simulink model "test_d_v_p"  (Simulink 6.2)
settings: Solver=ode45  StartTime=0.0  StopTime=30000  RelTol=1e-3
undefined symbols (not defined in the file or in its folder): ant_bits, blockCountBits, blockRowBits
libraries: xbsIndex_r3 x843, xps_library x50, casper_library x17
(part 2 of 6)

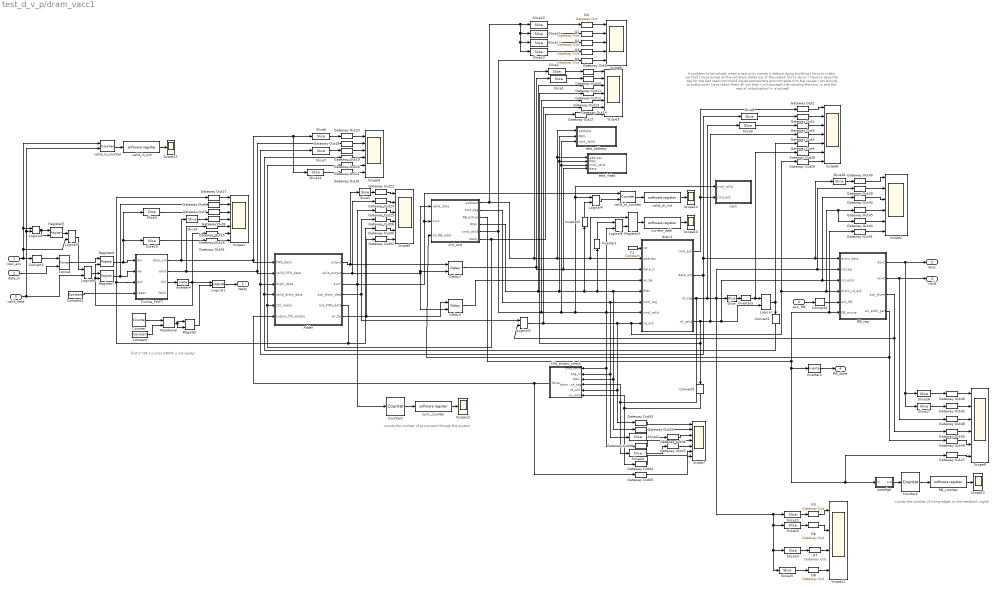
== system test_d_v_p/dram_vacc1 ==
  note: counts the number of rising edges on
      | the readback signal
  note: counts the number of syncs
      | sent through the system
  note: first 2^28-1 cycles DRAM
      | is not ready!
  note: A problem to be solved:
      | when a new sync comes in before doing anything I have to make sur
      | that I have acked all the old dram datas out of the output fifo
      | to do so: I have to save the tag for the last read command issued somewhere
      | and compare it to the values I am acking to make sure I have taken them all out
      | then I will proceed with sending the sync in and the rest of initialization!
      | it is solved!
  new_acc : Inport  Port=1  LatchInput=off
  data_in : Inport  Port=2  LatchInput=off
  valid_data : Inport  Port=3  LatchInput=off
  ack_RB : Inport  Port=4  LatchInput=off
  Adder : Subsystem
  C1 : xbsIndex_r3/Constant  const=0  equ=P=C  arith_type=Boolean  n_bits=1  bin_pt=0  opselect=C  inp2=PCIN>>17  opr=+  inp1=P  carry=CIN  iostate=0  explicit_period=on  period=1  dbl_ovrd=off
  Concat : xbsIndex_r3/Concat  num_inputs=2  explicit_period=off  period=1  dbl_ovrd=off
  Constant : xbsIndex_r3/Constant  const=2^28-1  equ=P=C  arith_type=Unsigned  n_bits=28  bin_pt=0  opselect=C  inp2=PCIN>>17  opr=+  inp1=P  carry=CIN  iostate=0  explicit_period=on  period=1  dbl_ovrd=off
  Constant1 : xbsIndex_r3/Constant  const=0  equ=P=C  arith_type=Boolean  n_bits=28  bin_pt=0  opselect=C  inp2=PCIN>>17  opr=+  inp1=P  carry=CIN  iostate=0  explicit_period=on  period=1  dbl_ovrd=off
  Convert1 : xbsIndex_r3/Convert  Orientation=down  arith_type=Boolean  n_bits=31  bin_pt=0  quantization=Truncate  overflow=Wrap  latency=0  explicit_period=off  period=1  dbl_ovrd=off  show_param=off  inserted_by_tool=off  pipeline=off
      settings: xl_area=[0, 0, 0, 0, 0, 0, 0]
  Convert2 : xbsIndex_r3/Convert  arith_type=Unsigned  n_bits=1  bin_pt=0  quantization=Truncate  overflow=Wrap  latency=0  explicit_period=off  period=1  dbl_ovrd=off  show_param=off  inserted_by_tool=off  pipeline=off
      settings: xl_area=[0, 0, 0, 0, 0, 0, 0]
  Convert3 : xbsIndex_r3/Convert  Orientation=down  arith_type=Boolean  n_bits=31  bin_pt=0  quantization=Truncate  overflow=Wrap  latency=0  explicit_period=off  period=1  dbl_ovrd=off  show_param=off  inserted_by_tool=off  pipeline=off
      settings: xl_area=[0, 0, 0, 0, 0, 0, 0]
  Convert4 : xbsIndex_r3/Convert  arith_type=Boolean  n_bits=31  bin_pt=0  quantization=Truncate  overflow=Wrap  latency=0  explicit_period=off  period=1  dbl_ovrd=off  show_param=off  inserted_by_tool=off  pipeline=off
      settings: xl_area=[0, 0, 0, 0, 0, 0, 0]
  Counter : xbsIndex_r3/Counter  cnt_type=Free Running  n_bits=28  bin_pt=0  arith_type=Unsigned  start_count=0  cnt_to=Inf  cnt_by_val=1  operation=Up  explicit_period=off  period=1  load_pin=off  rst=off  en=off  dbl_ovrd=off  show_param=off  use_rpm=on  gen_core=off
      settings: xl_area=[0, 0, 0, 0, 0, 0, 0]
  Counter1 : xbsIndex_r3/Counter  cnt_type=Free Running  n_bits=10  bin_pt=0  arith_type=Unsigned  start_count=0  cnt_to=Inf  cnt_by_val=1  operation=Up  explicit_period=off  period=1  load_pin=off  rst=off  en=on  dbl_ovrd=off  show_param=off  use_rpm=on  gen_core=off
      settings: xl_area=[0, 0, 0, 0, 0, 0, 0]
  Counter2 : xbsIndex_r3/Counter  cnt_type=Free Running  n_bits=10  bin_pt=0  arith_type=Unsigned  start_count=0  cnt_to=Inf  cnt_by_val=1  operation=Up  explicit_period=off  period=1  load_pin=off  rst=off  en=on  dbl_ovrd=off  show_param=off  use_rpm=on  gen_core=off
      settings: xl_area=[0, 0, 0, 0, 0, 0, 0]
  Delay1 : xbsIndex_r3/Delay  latency=1  reg_retiming=off  explicit_period=on  period=1  en=on  accept_only_valid=off  init_zero=on  dbl_ovrd=off  show_param=off
      settings: xl_area=[0, 0, 0, 0, 0, 0, 0]
  Delay2 : xbsIndex_r3/Delay  latency=1  reg_retiming=off  explicit_period=on  period=1  en=on  accept_only_valid=off  init_zero=on  dbl_ovrd=off  show_param=off
      settings: xl_area=[0, 0, 0, 0, 0, 0, 0]
  G{0..8} (9 alike) : xbsIndex_r3/Gateway Out  output_type=Double  nbits=8  bin_pt=6  arith_type=Boolean  quantization=Truncate  overflow=Wrap  hdl_port=off  timing_constraint=None  locs_specified=off  LOCs={}  needs_fixed_name=off  show_param=off
      settings: xl_area=[0, 0, 0, 0, 0, 0, 0]
  Gateway Out{1..52} (52 alike) : xbsIndex_r3/Gateway Out  output_type=Double  nbits=8  bin_pt=6  arith_type=Boolean  quantization=Truncate  overflow=Wrap  hdl_port=off  timing_constraint=None  locs_specified=off  LOCs={}  needs_fixed_name=off  show_param=off
      settings: xl_area=[0, 0, 0, 0, 0, 0, 0]
  Inverter1 : xbsIndex_r3/Inverter  Orientation=up  latency=0  explicit_period=off  period=1  en=off  dbl_ovrd=off  show_param=off
      settings: xl_area=[0, 0, 0, 0, 0, 0, 0]
  Inverter2 : xbsIndex_r3/Inverter  latency=0  explicit_period=off  period=1  en=off  dbl_ovrd=off  show_param=off
      settings: xl_area=[0, 0, 0, 0, 0, 0, 0]
  Inverter3 : xbsIndex_r3/Inverter  latency=0  explicit_period=off  period=1  en=off  dbl_ovrd=off  show_param=off
      settings: xl_area=[0, 0, 0, 0, 0, 0, 0]
  Inverter4 : xbsIndex_r3/Inverter  latency=0  explicit_period=off  period=1  en=off  dbl_ovrd=off  show_param=off
      settings: xl_area=[0, 0, 0, 0, 0, 0, 0]
  Inverter5 : xbsIndex_r3/Inverter  Orientation=up  latency=0  explicit_period=off  period=1  en=off  dbl_ovrd=off  show_param=off
      settings: xl_area=[0, 0, 0, 0, 0, 0, 0]
  Logical{,1,3..4,6,8} (6 alike) : xbsIndex_r3/Logical  logical_function=AND  inputs=2  precision=Full  arith_type=Unsigned  n_bits=8  bin_pt=2  align_bp=on  latency=0  explicit_period=off  period=1  en=off  dbl_ovrd=off  show_param=off
      settings: xl_area=[0, 0, 0, 0, 0, 0, 0]
  Logical2 : xbsIndex_r3/Logical  logical_function=OR  inputs=2  precision=Full  arith_type=Unsigned  n_bits=8  bin_pt=2  align_bp=on  latency=0  explicit_period=off  period=1  en=off  dbl_ovrd=off  show_param=off
      settings: xl_area=[0, 0, 0, 0, 0, 0, 0]
  Logical7 : xbsIndex_r3/Logical  logical_function=OR  inputs=2  precision=Full  arith_type=Unsigned  n_bits=8  bin_pt=2  align_bp=on  latency=0  explicit_period=off  period=1  en=off  dbl_ovrd=off  show_param=off
      settings: xl_area=[0, 0, 0, 0, 0, 0, 0]
  RB_counter : xps_library/software register  Tag=xps:sw_reg  io_dir=To Processor  arith_type=Unsigned  bitwidth=32  bin_pt=0  sample_period=1  gw_name=test_d_v_p_dram_vacc1_RB_counter_user_data_in
  RB_reg : Subsystem
  Register{,2,5..7} (5 alike) : xbsIndex_r3/Register  init=0  reg_only_valid=off  explicit_period=off  period=1  rst=off  en=on  out_en=off  dbl_ovrd=off  show_param=off
      settings: xl_area=[0, 0, 0, 0, 0, 0, 0]
  Relational : xbsIndex_r3/Relational  mode=a=b  latency=1  explicit_period=off  period=1  en=off  dbl_ovrd=off  show_param=off
      settings: xl_area=[0, 0, 0, 0, 0, 0, 0]
  Scope{1,3,7..8} (4 alike) : Scope  NumInputPorts=7
      Scope1 settings: TimeRange=30000  YMin=0~0~0.95~0.95~0~0.95~-1  YMax=1~1~1.05~1.05~1~1.05~1  SaveName=ScopeData7
      Scope3 settings: YMin=0~0~0~0~0~0~0  YMax=150~2500~1~1~1~1~1  SaveName=ScopeData6
      Scope7 settings: YMin=0~0~0~0~0~0.95~0  YMax=1~1100~7500~1~1~1.05~1  SaveName=ScopeData17
      Scope8 settings: YMin=0~0~2.68438e+008~0~0~0~0  YMax=1~11000~2.68439e+008~1~1~1~1  SaveName=ScopeData19
  Scope{10,12..15} (5 alike) : Scope
      Scope10 settings: YMin=0  YMax=100  SaveName=ScopeData27
      Scope12 settings: YMin=0  YMax=100  SaveName=ScopeData32
      Scope13 settings: YMin=0  YMax=100  SaveName=ScopeData33
      Scope14 settings: YMin=0  YMax=100  SaveName=ScopeData21
      Scope15 settings: YMin=0  YMax=100  SaveName=ScopeData24
  Scope11 : Scope  NumInputPorts=4
      settings: YMin=0~0.95~-1~1.9  YMax=120~1.05~1~2.1  SaveName=ScopeData28
  Scope{2,4..5,9} (4 alike) : Scope  NumInputPorts=6
      Scope2 settings: YMin=2.5~5e+008~0~0~0~0.95  YMax=12.5~2.75e+009~1~1~1~1.05  SaveName=ScopeData22
      Scope4 settings: YMin=0.95~0.95~-1~-1~0.95~-1  YMax=1.05~1.05~1~1~1.05~1  SaveName=ScopeData8
      Scope5 settings: YMin=0~0~-1~0~0~-5  YMax=250~1~1~1~1~5  SaveName=ScopeData9
      Scope9 settings: YMin=1.9~1.9~-1~0~-1~0.95  YMax=2.1~2.1~1~1~1~1.05  SaveName=ScopeData23
  Scope6 : Scope  NumInputPorts=5
      settings: YMin=0~0~0~0~0  YMax=200~4000~1~1~1  SaveName=ScopeData14
  Slice : xbsIndex_r3/Slice  mode=Upper Bit Location + Width  nbits=1  bit1=0  base1=MSB of Input  bit0=0  base0=LSB of Input  boolean_output=off  explicit_period=off  period=1  dbl_ovrd=off
  Slice{1,3..8,16..18} (10 alike) : xbsIndex_r3/Slice  mode=Lower Bit Location + Width  nbits=32  bit1=0  base1=MSB of Input  bit0=0  base0=LSB of Input  boolean_output=off  explicit_period=off  period=1  dbl_ovrd=off
  Slice{2,10,20,22} (4 alike) : xbsIndex_r3/Slice  mode=Lower Bit Location + Width  nbits=8  bit1=0  base1=MSB of Input  bit0=5  base0=LSB of Input  boolean_output=off  explicit_period=off  period=1  dbl_ovrd=off
  Slice11 : xbsIndex_r3/Slice  mode=Lower Bit Location + Width  nbits=14  bit1=0  base1=MSB of Input  bit0=14  base0=LSB of Input  boolean_output=off  explicit_period=off  period=1  dbl_ovrd=off
  Slice12 : xbsIndex_r3/Slice  mode=Lower Bit Location + Width  nbits=1  bit1=0  base1=MSB of Input  bit0=13  base0=LSB of Input  boolean_output=off  explicit_period=off  period=1  dbl_ovrd=off
  Slice13 : xbsIndex_r3/Slice  mode=Lower Bit Location + Width  nbits=2  bit1=0  base1=MSB of Input  bit0=28  base0=LSB of Input  boolean_output=off  explicit_period=off  period=1  dbl_ovrd=off
  Slice14 : xbsIndex_r3/Slice  mode=Upper Bit Location + Width  nbits=1  bit1=0  base1=MSB of Input  bit0=0  base0=LSB of Input  boolean_output=off  explicit_period=off  period=1  dbl_ovrd=off
  Slice19 : xbsIndex_r3/Slice  mode=Upper Bit Location + Width  nbits=1  bit1=0  base1=MSB of Input  bit0=0  base0=LSB of Input  boolean_output=off  explicit_period=off  period=1  dbl_ovrd=off
  Slice21 : xbsIndex_r3/Slice  mode=Lower Bit Location + Width  nbits=8  bit1=0  base1=MSB of Input  bit0=6  base0=LSB of Input  boolean_output=off  explicit_period=off  period=1  dbl_ovrd=off
  Slice23 : xbsIndex_r3/Slice  mode=Lower Bit Location + Width  nbits=14  bit1=0  base1=MSB of Input  bit0=15  base0=LSB of Input  boolean_output=off  explicit_period=off  period=1  dbl_ovrd=off
  Slice24 : xbsIndex_r3/Slice  mode=Lower Bit Location + Width  nbits=1  bit1=0  base1=MSB of Input  bit0=14  base0=LSB of Input  boolean_output=off  explicit_period=off  period=1  dbl_ovrd=off
  Slice25 : xbsIndex_r3/Slice  mode=Lower Bit Location + Width  nbits=2  bit1=0  base1=MSB of Input  bit0=29  base0=LSB of Input  boolean_output=off  explicit_period=off  period=1  dbl_ovrd=off
  Slice9 : xbsIndex_r3/Slice  mode=Lower Bit Location + Width  nbits=31  bit1=0  base1=MSB of Input  bit0=0  base0=LSB of Input  boolean_output=off  explicit_period=off  period=1  dbl_ovrd=off
  Trickle_FWFT : Subsystem  mask{depth=512}
      mask init:
      | cursys = gcb ; 
      | set_param([cursys, '/FIFO'], 'depth', depth);
      mask StyleString: popup(16|32|64|128|256|512|1K|2K|4K|8K|16K|32K|64K)
  cack : Subsystem
  ctrl_unit : Subsystem  mask{burst_length=valid_length, acc_length=acc_length}
      mask prompts: burst_length "Burst Length?"; acc_length "Accumulation length?"
  current_addr : xps_library/software register  Tag=xps:sw_reg  io_dir=To Processor  arith_type=Unsigned  bitwidth=32  bin_pt=0  sample_period=1  gw_name=test_d_v_p_dram_vacc1_current_addr_user_data_in
  dram1 : Subsystem  Tag=xps:dram  AncestorBlock=xps_library/dram  mask(dram){dimm=1, arith_type=Unsigned, bin_pt=0, ip_clock=200, sample_period=1, use_sim=on, bank_mgt=on, wide_data=off, half_burst=off, shared=on}
      mask prompts: arith_type "Data Type"; bin_pt "Data binary point"; ip_clock "Datapath clock rate (MHz)"; sample_period "Sample period"; use_sim "Simulate DRAM using ModelSim"; bank_mgt "Enable bank management"; wide_data "Use wide data bus (288 bits)"; half_burst "Use half-burst"; shared "Share with PowerPC"
      mask help:
      | Interface to 1GB DDR2 DIMMs on BEE2.
      |
      | To simulate using ModelSim, place a ModelSim block named 'ModelSim' (case-sensitive) in the top level of the design.
      mask init:
      | dram_mask;
      mask StyleString: popup(1|2|3|4),popup(Boolean|Unsigned|Signed  (2's comp)),edit,edit,edit,checkbox,checkbox,checkbox,checkbox,checkbox
      mask CallbackString:
      | |||||||myname=gcb;
      | if strcmp(get_param(myname, 'wide_data'), 'off')
      |     set_param(myname, 'MaskEnables', {'on','on','on','on','on','on','on','on','on','on'});
      | else
      |     set_param(myname, 'half_burst', 'off');
      |     set_param(myname, 'MaskEnables', {'on','on','on','on','on','on','on','on','off','on'});
      | end||
  fifo_empty_check : Subsystem  Orientation=left
  posedge : Subsystem
  sync_counter : xps_library/software register  Tag=xps:sw_reg  io_dir=To Processor  arith_type=Unsigned  bitwidth=32  bin_pt=0  sample_period=1  gw_name=test_d_v_p_dram_vacc1_sync_counter_user_data_in
  test_address : Subsystem
  test_index : Subsystem
  valid_dr_cnt : xps_library/software register  Tag=xps:sw_reg  io_dir=To Processor  arith_type=Unsigned  bitwidth=32  bin_pt=0  sample_period=1  gw_name=test_d_v_p_dram_vacc1_valid_dr_cnt_user_data_in
  valid_dr_counter : xbsIndex_r3/Counter  cnt_type=Count Limited  n_bits=32  bin_pt=0  arith_type=Unsigned  start_count=0  cnt_to=Inf  cnt_by_val=1  operation=Up  explicit_period=off  period=1  load_pin=off  rst=on  en=on  dbl_ovrd=off  show_param=off  use_rpm=on  gen_core=off
      settings: xl_area=[0, 0, 0, 0, 0, 0, 0]
  valid_in_cnt : xps_library/software register  Tag=xps:sw_reg  io_dir=To Processor  arith_type=Unsigned  bitwidth=32  bin_pt=0  sample_period=1  gw_name=test_d_v_p_dram_vacc1_valid_in_cnt_user_data_in
  valid_in_counter : xbsIndex_r3/Counter  cnt_type=Count Limited  n_bits=32  bin_pt=0  arith_type=Unsigned  start_count=0  cnt_to=Inf  cnt_by_val=1  operation=Up  explicit_period=off  period=1  load_pin=off  rst=on  en=on  dbl_ovrd=off  show_param=off  use_rpm=on  gen_core=off
      settings: xl_area=[0, 0, 0, 0, 0, 0, 0]
  ready : Outport
  dout : Outport  Port=2
  valid : Outport  Port=3
  RB_done : Outport  Port=4
  wires:
  Convert4/1 -> RB_reg/5(ack_RB)
  Inverter3/1 -> Gateway Out28/1, Logical/1
  ack_RB/1 -> Convert4/1
  ctrl_unit/5(cmd_valid) -> G4/1, Gateway Out13/1, Logical6/2, Gateway Out38/1, fifo_empty_check/1(cmd_valid), dram1/7(cmd_valid), cack/1(cmd_valid), Logical4/1, test_address/3(cmd_valid), test_index/3(cmd_valid)
  Inverter2/1 -> RB_done/1
  posedge/1(out) -> Counter2/1
  RB_counter/1 -> Scope13/1
  Counter2/1 -> RB_counter/1
  sync_counter/1 -> Scope12/1
  Counter1/1 -> sync_counter/1
  Inverter4/1 -> Logical1/1, Gateway Out16/1, Register7/2, Register6/2
  G8/1 -> Scope11/4
  G7/1 -> Scope11/3
  G6/1 -> Scope11/2
  G5/1 -> Scope11/1
  Slice25/1 -> G8/1
  Slice24/1 -> G7/1
  Slice23/1 -> G6/1
  Slice21/1 -> G5/1
  Slice20/1 -> Gateway Out37/1
  Slice22/1 -> Gateway Out36/1
  current_addr/1 -> Scope10/1
  Inverter1/1 -> Logical6/1
  Logical6/1 -> Register2/2
  Register2/1 -> current_addr/1
  Slice19/1 -> Gateway Out51/1
  Gateway Out51/1 -> Scope1/7
  Register7/1 -> Gateway Out6/1, Trickle_FWFT/2(we)
  Register/1 -> Logical1/2
  Relational/1 -> Register/2, Register/1
  Constant/1 -> Relational/2
  Counter/1 -> Relational/1
  Logical1/1 -> ready/1
  Gateway Out47/1 -> Scope9/6
  Slice18/1 -> Gateway Out40/1
  Slice17/1 -> Gateway Out42/1
  Slice16/1 -> Gateway Out46/1
  Convert3/1 -> Gateway Out34/1, fifo_empty_check/6(rd_valid)
  Gateway Out49/1 -> Scope9/5
  Gateway Out50/1 -> Scope9/4
  Gateway Out48/1 -> Scope9/3
  Gateway Out42/1 -> Scope9/2
  Gateway Out46/1 -> Scope9/1
  Gateway Out41/1 -> Scope2/6
  Gateway Out44/1 -> Scope2/5
  Gateway Out45/1 -> Scope2/4
  Gateway Out43/1 -> Scope2/3
  Gateway Out39/1 -> Scope2/2
  Gateway Out40/1 -> Scope2/1
  Logical2/1 -> Gateway Out14/1, Gateway Out44/1, Gateway Out45/1, RB_reg/4(dram_rd_ack), Gateway Out29/1, dram1/8(rd_ack), Gateway Out33/1, fifo_empty_check/5(rd_ack)
  ctrl_unit/3(RB_active) -> Inverter2/1, posedge/1(in), Gateway Out47/1, RB_reg/6(RB_active), Gateway Out41/1
  RB_reg/4(en_addr_gen) -> Gateway Out49/1, ctrl_unit/3(en_RB_addr)
  RB_reg/3(ack_dram) -> Logical2/2, Gateway Out50/1
  RB_reg/2(valid) -> valid/1, Gateway Out48/1
  RB_reg/1(dout) -> Slice17/1, Slice16/1, dout/1
  Gateway Out29/1 -> Scope8/7
  Gateway Out28/1 -> Scope8/6
  Gateway Out4/1 -> Scope8/5
  Gateway Out5/1 -> Scope8/4
  Gateway Out3/1 -> Scope8/3
  Gateway Out1/1 -> Scope8/2
  Gateway Out2/1 -> Scope8/1
  Gateway Out35/1 -> Scope7/7
  Gateway Out34/1 -> Scope7/6
  Gateway Out38/1 -> Scope7/4
  Gateway Out37/1 -> Scope7/5
  Gateway Out36/1 -> Scope7/3
  Gateway Out32/1 -> Scope7/2
  Gateway Out33/1 -> Scope7/1
  fifo_empty_check/1(done) -> Gateway Out35/1, Adder/6(output_fifo_empty)
  Delay1/1 -> Slice1/1, dram1/3(data_in), test_index/4(data)
  Slice14/1 -> Gateway Out31/1
  Gateway Out31/1 -> Scope4/6
  G4/1 -> Scope6/5
  G3/1 -> Scope6/4
  G2/1 -> Scope6/3
  G1/1 -> Scope6/2
  G0/1 -> Scope6/1
  Slice13/1 -> G3/1
  Slice12/1 -> G2/1
  Slice11/1 -> G1/1
  Slice10/1 -> G0/1
  Gateway Out30/1 -> Scope5/5
  Adder/5(ack_FIFO_data) -> Gateway Out30/1, Gateway Out17/1, Trickle_FWFT/3(ack)
  Slice9/1 -> Gateway Out3/1
  Slice8/1 -> Gateway Out1/1
  Gateway Out27/1 -> Scope3/7
  Slice7/1 -> Gateway Out19/1
  Slice6/1 -> Gateway Out23/1
  Slice5/1 -> Gateway Out22/1
  Convert1/1 -> Adder/4(valid_dram_data), Gateway Out20/1
  Slice4/1 -> Gateway Out8/1
  Slice3/1 -> Gateway Out7/1
  Gateway Out26/1 -> Scope5/4
  Gateway Out25/1 -> Scope5/3
  Gateway Out24/1 -> Scope5/2
  Gateway Out22/1 -> Scope5/1
  Gateway Out21/1 -> Scope4/5
  Gateway Out20/1 -> Scope4/4
  Gateway Out19/1 -> Scope4/3
  Gateway Out18/1 -> Scope4/2
  Gateway Out23/1 -> Scope4/1
  Gateway Out16/1 -> Scope1/6
  Gateway Out15/1 -> Scope1/5
  Gateway Out8/1 -> Scope1/4
  Gateway Out7/1 -> Scope1/3
  Gateway Out6/1 -> Scope1/2
  Gateway Out17/1 -> Scope1/1
  Slice2/1 -> Gateway Out9/1
  Slice1/1 -> Gateway Out10/1
  Gateway Out14/1 -> Scope3/6
  Gateway Out13/1 -> Scope3/5
  Gateway Out12/1 -> Scope3/4
  Gateway Out11/1 -> Scope3/3
  Gateway Out10/1 -> Scope3/2
  Gateway Out9/1 -> Scope3/1
  Register6/1 -> Slice19/1, Slice3/1, Trickle_FWFT/1(din)
  Trickle_FWFT/3(full) -> Inverter4/1
  ctrl_unit/2(cmd_tag) -> Slice22/1, fifo_empty_check/2(tag_in), dram1/6(cmd_tag)
  dram1/1(cmd_ack) -> Gateway Out2/1, cack/2(cmd_ack)
  Adder/3(sync) -> Counter1/1, ctrl_unit/2(sync), valid_dr_counter/1, Gateway Out25/1
  Adder/2(valid_output) -> Gateway Out24/1, Delay1/2, ctrl_unit/1(valid_data), Delay2/2
  ctrl_unit/6(ready) -> Gateway Out27/1, Adder/5(ctrl_ready), Gateway Out21/1
  Logical/1 -> Convert1/1, Gateway Out4/1
  dram1/4(rd_valid) -> Convert3/1, Gateway Out12/1, RB_reg/3(rd_valid), Gateway Out43/1, Logical/2, Gateway Out5/1
  Slice/1 -> Inverter3/1
  dram1/3(rd_tag) -> Slice20/1, fifo_empty_check/4(dram_data_tag), RB_reg/2(rd_tag), Gateway Out39/1, Slice/1, Slice24/1, Slice25/1, Slice23/1, Slice21/1, Slice9/1
  dram1/2(data_out) -> RB_reg/1(dram_data), Slice18/1, Slice8/1, Adder/3(dram_data), Slice7/1
  Adder/1(output) -> Delay1/1, Slice5/1
  C1/1 -> dram1/1(rst)
  ctrl_unit/4(RWn) -> Gateway Out11/1, Inverter1/1, Gateway Out32/1, fifo_empty_check/3(RWn), dram1/5(RWn), Inverter5/1, test_address/2(RWn), test_index/2(RWn)
  ctrl_unit/1(address) -> Slice2/1, Register2/1, dram1/2(address), test_address/1(address), test_index/1(address), Slice12/1, Slice13/1, Slice11/1, Slice10/1
  Trickle_FWFT/2(valid) -> Adder/2(valid_FIFO_data), Gateway Out18/1, Gateway Out15/1
  Trickle_FWFT/1(data_out) -> Slice4/1, Slice14/1, Slice6/1, Adder/1(FIFO_data)
  Adder/4(ack_dram_data) -> Logical2/1, Gateway Out26/1
  new_acc/1 -> Convert2/1, Logical7/2, Logical3/1, valid_in_counter/1
  data_in/1 -> Concat/2
  valid_data/1 -> Logical8/2, Logical3/2, valid_in_counter/2
  Convert2/1 -> Concat/1
  Register5/1 -> Logical7/1
  Logical7/1 -> Logical8/1
  Logical3/1 -> Register5/1, Register5/2
  Concat/1 -> Register6/1
  Logical8/1 -> Register7/1
  Constant1/1 -> Trickle_FWFT/4(reset)
  Logical4/1 -> valid_dr_counter/2
  valid_dr_cnt/1 -> Scope14/1
  valid_dr_counter/1 -> valid_dr_cnt/1
  Inverter5/1 -> Logical4/2
  valid_in_cnt/1 -> Scope15/1
  valid_in_counter/1 -> valid_in_cnt/1
  Adder/6(wr_be) -> Delay2/1, Gateway Out52/1
  Delay2/1 -> dram1/4(wr_be)
  Gateway Out52/1 -> Scope5/6

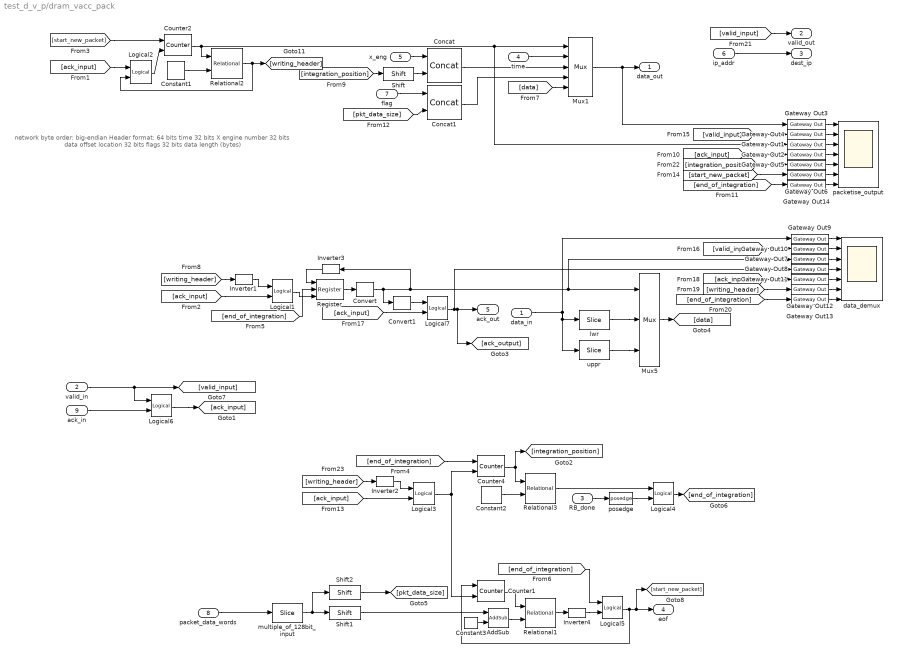
== system test_d_v_p/dram_vacc_pack ==
  note: network byte order: big-endian
      |
      | Header format:
      | 64 bits time
      | 32 bits X engine number
      | 32 bits data offset location
      | 32 bits flags
      | 32 bits data length (bytes)
  data_in : Inport  Port=1  LatchInput=off
  valid_in : Inport  Port=2  LatchInput=off
  RB_done : Inport  Port=3  LatchInput=off
  time : Inport  Port=4  LatchInput=off
  x_eng : Inport  Port=5  LatchInput=off
  ip_addr : Inport  Port=6  LatchInput=off
  flag : Inport  Port=7  LatchInput=off
  packet_data_words : Inport  Port=8  LatchInput=off
  ack_in : Inport  Port=9  LatchInput=off
  AddSub : xbsIndex_r3/AddSub  mode=Subtraction  precision=Full  arith_type=Unsigned  n_bits=8  bin_pt=2  quantization=Truncate  overflow=Wrap  latency=0  explicit_period=on  period=1  use_carryin=off  use_carryout=off  en=off  dbl_ovrd=off  show_param=off  use_core=on  pipeline=off  use_rpm=on  gen_core=off
      settings: xl_area=[0, 0, 0, 0, 0, 0, 0]
  Concat : xbsIndex_r3/Concat  num_inputs=2  explicit_period=off  period=1  dbl_ovrd=off
  Concat1 : xbsIndex_r3/Concat  num_inputs=2  explicit_period=off  period=1  dbl_ovrd=off
  Constant1 : xbsIndex_r3/Constant  const=2  equ=P=C  arith_type=Unsigned  n_bits=2  bin_pt=0  opselect=C  inp2=PCIN>>17  opr=+  inp1=P  carry=CIN  iostate=0  explicit_period=off  period=1  dbl_ovrd=off
  Constant2 : xbsIndex_r3/Constant  const=2*vector_len-1  equ=P=C  arith_type=Unsigned  n_bits=32  bin_pt=0  opselect=C  inp2=PCIN>>17  opr=+  inp1=P  carry=CIN  iostate=0  explicit_period=off  period=1  dbl_ovrd=off
  Constant3 : xbsIndex_r3/Constant  const=2  equ=P=C  arith_type=Unsigned  n_bits=32  bin_pt=0  opselect=C  inp2=PCIN>>17  opr=+  inp1=P  carry=CIN  iostate=0  explicit_period=off  period=1  dbl_ovrd=off
  Convert : xbsIndex_r3/Convert  arith_type=Unsigned  n_bits=1  bin_pt=0  quantization=Truncate  overflow=Wrap  latency=0  explicit_period=off  period=1  dbl_ovrd=off  show_param=off  inserted_by_tool=off  pipeline=off
      settings: xl_area=[0, 0, 0, 0, 0, 0, 0]
  Convert1 : xbsIndex_r3/Convert  arith_type=Boolean  n_bits=1  bin_pt=0  quantization=Truncate  overflow=Wrap  latency=0  explicit_period=off  period=1  dbl_ovrd=off  show_param=off  inserted_by_tool=off  pipeline=off
      settings: xl_area=[0, 0, 0, 0, 0, 0, 0]
  Counter1 : xbsIndex_r3/Counter  cnt_type=Free Running  n_bits=32  bin_pt=0  arith_type=Unsigned  start_count=0  cnt_to=1023  cnt_by_val=1  operation=Up  explicit_period=on  period=1  load_pin=off  rst=on  en=on  dbl_ovrd=off  show_param=off  use_rpm=on  gen_core=off
      settings: xl_area=[0, 0, 0, 0, 0, 0, 0]
  Counter2 : xbsIndex_r3/Counter  cnt_type=Free Running  n_bits=2  bin_pt=0  arith_type=Unsigned  start_count=0  cnt_to=1023  cnt_by_val=1  operation=Up  explicit_period=on  period=1  load_pin=off  rst=on  en=on  dbl_ovrd=off  show_param=off  use_rpm=on  gen_core=off
      settings: xl_area=[0, 0, 0, 0, 0, 0, 0]
  Counter4 : xbsIndex_r3/Counter  cnt_type=Free Running  n_bits=32  bin_pt=0  arith_type=Unsigned  start_count=0  cnt_to=1023  cnt_by_val=1  operation=Up  explicit_period=on  period=1  load_pin=off  rst=on  en=on  dbl_ovrd=off  show_param=off  use_rpm=on  gen_core=off
      settings: xl_area=[0, 0, 0, 0, 0, 0, 0]
  Gateway Out{1..14} (14 alike) : xbsIndex_r3/Gateway Out  output_type=Double  nbits=8  bin_pt=6  arith_type=Boolean  quantization=Truncate  overflow=Wrap  hdl_port=on  timing_constraint=None  locs_specified=off  LOCs={}  needs_fixed_name=off  show_param=off
      settings: xl_area=[0, 0, 0, 0, 0, 0, 0]
  Inverter1 : xbsIndex_r3/Inverter  latency=0  explicit_period=off  period=1  en=off  dbl_ovrd=off  show_param=off
      settings: xl_area=[0, 0, 0, 0, 0, 0, 0]
  Inverter2 : xbsIndex_r3/Inverter  latency=0  explicit_period=off  period=1  en=off  dbl_ovrd=off  show_param=off
      settings: xl_area=[0, 0, 0, 0, 0, 0, 0]
  Inverter3 : xbsIndex_r3/Inverter  Orientation=left  latency=0  explicit_period=on  period=1  en=off  dbl_ovrd=off  show_param=off
      settings: xl_area=[0, 0, 0, 0, 0, 0, 0]
  Inverter4 : xbsIndex_r3/Inverter  latency=0  explicit_period=off  period=1  en=off  dbl_ovrd=off  show_param=off
      settings: xl_area=[0, 0, 0, 0, 0, 0, 0]
  Logical{1..3,6..7} (5 alike) : xbsIndex_r3/Logical  logical_function=AND  inputs=2  precision=Full  arith_type=Unsigned  n_bits=8  bin_pt=2  align_bp=on  latency=0  explicit_period=off  period=1  en=off  dbl_ovrd=off  show_param=off
      settings: xl_area=[0, 0, 0, 0, 0, 0, 0]
  Logical4 : xbsIndex_r3/Logical  logical_function=OR  inputs=2  precision=Full  arith_type=Unsigned  n_bits=8  bin_pt=2  align_bp=on  latency=0  explicit_period=off  period=1  en=off  dbl_ovrd=off  show_param=off
      settings: xl_area=[0, 0, 0, 0, 0, 0, 0]
  Logical5 : xbsIndex_r3/Logical  logical_function=OR  inputs=2  precision=Full  arith_type=Unsigned  n_bits=8  bin_pt=2  align_bp=on  latency=0  explicit_period=off  period=1  en=off  dbl_ovrd=off  show_param=off
      settings: xl_area=[0, 0, 0, 0, 0, 0, 0]
  Mux1 : xbsIndex_r3/Mux  inputs=4  precision=Full  arith_type="Signed  (2's comp)"  n_bits=8  bin_pt=2  quantization=Truncate  overflow=Wrap  latency=0  explicit_period=off  period=1  en=off  dbl_ovrd=off  show_param=off  mux_type=off  use_rpm=off  gen_core=off
      settings: xl_area=[0, 0, 0, 0, 0, 0, 0]
  Mux5 : xbsIndex_r3/Mux  inputs=2  precision=Full  arith_type="Signed  (2's comp)"  n_bits=8  bin_pt=2  quantization=Truncate  overflow=Wrap  latency=0  explicit_period=on  period=1  en=off  dbl_ovrd=off  show_param=off  mux_type=off  use_rpm=off  gen_core=off
      settings: xl_area=[0, 0, 0, 0, 0, 0, 0]
  Register : xbsIndex_r3/Register  init=0  reg_only_valid=off  explicit_period=on  period=1  rst=on  en=on  out_en=off  dbl_ovrd=off  show_param=off
      settings: xl_area=[0, 0, 0, 0, 0, 0, 0]
  Relational1 : xbsIndex_r3/Relational  mode=a<=b  latency=0  explicit_period=off  period=1  en=off  dbl_ovrd=off  show_param=off
      settings: xl_area=[0, 0, 0, 0, 0, 0, 0]
  Relational2 : xbsIndex_r3/Relational  mode=a<=b  latency=0  explicit_period=off  period=1  en=off  dbl_ovrd=off  show_param=off
      settings: xl_area=[0, 0, 0, 0, 0, 0, 0]
  Relational3 : xbsIndex_r3/Relational  mode=a>=b  latency=0  explicit_period=off  period=1  en=off  dbl_ovrd=off  show_param=off
      settings: xl_area=[0, 0, 0, 0, 0, 0, 0]
  Shift : xbsIndex_r3/Shift  shift_dir=Left  shift_bits=3  precision=Full  arith_type="Signed  (2's comp)"  n_bits=8  bin_pt=2  quantization=Truncate  overflow=Wrap  latency=0  explicit_period=off  period=1  en=off  dbl_ovrd=off  show_param=off
      settings: xl_area=[0, 0, 0, 0, 0, 0, 0]
  Shift1 : xbsIndex_r3/Shift  shift_dir=Left  shift_bits=1  precision=Full  arith_type="Signed  (2's comp)"  n_bits=8  bin_pt=2  quantization=Truncate  overflow=Wrap  latency=0  explicit_period=off  period=1  en=off  dbl_ovrd=off  show_param=off
      settings: xl_area=[0, 0, 0, 0, 0, 0, 0]
  Shift2 : xbsIndex_r3/Shift  shift_dir=Left  shift_bits=4  precision=Full  arith_type="Signed  (2's comp)"  n_bits=8  bin_pt=2  quantization=Truncate  overflow=Wrap  latency=0  explicit_period=off  period=1  en=off  dbl_ovrd=off  show_param=off
      settings: xl_area=[0, 0, 0, 0, 0, 0, 0]
  data_demux : Scope  NumInputPorts=7
      settings: YMin=410.4~-1~-1~-1~0~-5~-5  YMax=453.6~1~1~1~1~5~5  SaveName=ScopeData3
  lwr : xbsIndex_r3/Slice  mode=Lower Bit Location + Width  nbits=64  bit1=0  base1=MSB of Input  bit0=0  base0=LSB of Input  boolean_output=off  explicit_period=off  period=1  dbl_ovrd=off
  multiple_of_128bit_input : xbsIndex_r3/Slice  mode=Two Bit Locations  nbits=64  bit1=0  base1=MSB of Input  bit0=4  base0=LSB of Input  boolean_output=off  explicit_period=off  period=1  dbl_ovrd=off
  packetise_output : Scope  NumInputPorts=7
      settings: YMin=410.4~-1~-1~-1~0~-5~-5  YMax=453.6~1~1~1~1~5~5
  posedge : casper_library/Misc/posedge  Tag=Rising Edge Detector
  uppr : xbsIndex_r3/Slice  mode=Upper Bit Location + Width  nbits=64  bit1=0  base1=MSB of Input  bit0=0  base0=LSB of Input  boolean_output=off  explicit_period=off  period=1  dbl_ovrd=off
  data_out : Outport
  valid_out : Outport  Port=2
  dest_ip : Outport  Port=3
  eof : Outport  Port=4
  ack_out : Outport  Port=5
  wires:
  lwr/1 -> Mux5/2
  uppr/1 -> Mux5/3
  [ack_input] -> Logical1/2
  Counter1/1 -> Relational1/1
  Logical5/1 -> Counter1/1, eof/1, [start_new_packet]
  Constant1/1 -> Relational2/2
  Counter2/1 -> Relational2/1, Mux1/1, Gateway Out1/1
  time/1 -> Mux1/2
  Logical2/1 -> Counter2/2
  Relational2/1 -> Logical2/2, [writing_header]
  [ack_input] -> Logical2/1
  [start_new_packet] -> Counter2/1
  [end_of_integration] -> Counter4/1
  Counter4/1 -> [integration_position], Relational3/1
  Mux1/1 -> data_out/1, Gateway Out3/1
  Mux5/1 -> [data]
  [writing_header] -> Inverter1/1
  Inverter1/1 -> Logical1/1
  x_eng/1 -> Concat/1
  [integration_position] -> Shift/1
  Concat/1 -> Mux1/3
  valid_in/1 -> [valid_input], Logical6/1
  ip_addr/1 -> dest_ip/1
  flag/1 -> Concat1/1
  [pkt_data_size] -> Concat1/2
  Concat1/1 -> Mux1/4
  Logical3/1 -> Counter4/2, Counter1/2
  Gateway Out3/1 -> packetise_output/1
  Gateway Out4/1 -> packetise_output/2
  Gateway Out1/1 -> packetise_output/3
  Gateway Out2/1 -> packetise_output/4
  Gateway Out5/1 -> packetise_output/5
  Gateway Out6/1 -> packetise_output/6
  [data] -> Mux1/5
  Relational1/1 -> Inverter4/1
  [end_of_integration] -> Logical5/1
  Logical6/1 -> [ack_input]
  ack_in/1 -> Logical6/2
  [start_new_packet] -> Gateway Out6/1
  [valid_input] -> Gateway Out4/1
  Gateway Out9/1 -> data_demux/1
  Gateway Out10/1 -> data_demux/2
  Gateway Out7/1 -> data_demux/3
  Gateway Out8/1 -> data_demux/4
  Gateway Out11/1 -> data_demux/5
  Gateway Out12/1 -> data_demux/6
  [valid_input] -> Gateway Out10/1
  Register/1 -> Convert/1
  Inverter3/1 -> Register/1
  [ack_input] -> Logical7/2
  Logical7/1 -> Gateway Out8/1, ack_out/1, [ack_output]
  Convert1/1 -> Logical7/1
  [ack_input] -> Gateway Out11/1
  [writing_header] -> Gateway Out12/1
  Gateway Out13/1 -> data_demux/7
  [end_of_integration] -> Gateway Out13/1
  data_in/1 -> uppr/1, lwr/1, Gateway Out9/1
  [valid_input] -> valid_out/1
  Convert/1 -> Inverter3/1, Mux5/1, Gateway Out7/1, Convert1/1
  Constant2/1 -> Relational3/2
  Gateway Out14/1 -> packetise_output/7
  [end_of_integration] -> Gateway Out14/1
  Shift/1 -> Concat/2
  Logical4/1 -> [end_of_integration]
  Relational3/1 -> Logical4/1
  RB_done/1 -> posedge/1
  posedge/1 -> Logical4/2
  [integration_position] -> Gateway Out5/1
  Logical1/1 -> Register/3
  [end_of_integration] -> Register/2
  [ack_input] -> Logical3/2
  [writing_header] -> Inverter2/1
  Inverter2/1 -> Logical3/1
  Inverter4/1 -> Logical5/2
  packet_data_words/1 -> multiple_of_128bit_input/1
  multiple_of_128bit_input/1 -> Shift1/1, Shift2/1
  Shift1/1 -> AddSub/1
  AddSub/1 -> Relational1/2
  Constant3/1 -> AddSub/2
  Shift2/1 -> [pkt_data_size]
  [ack_input] -> Gateway Out2/1

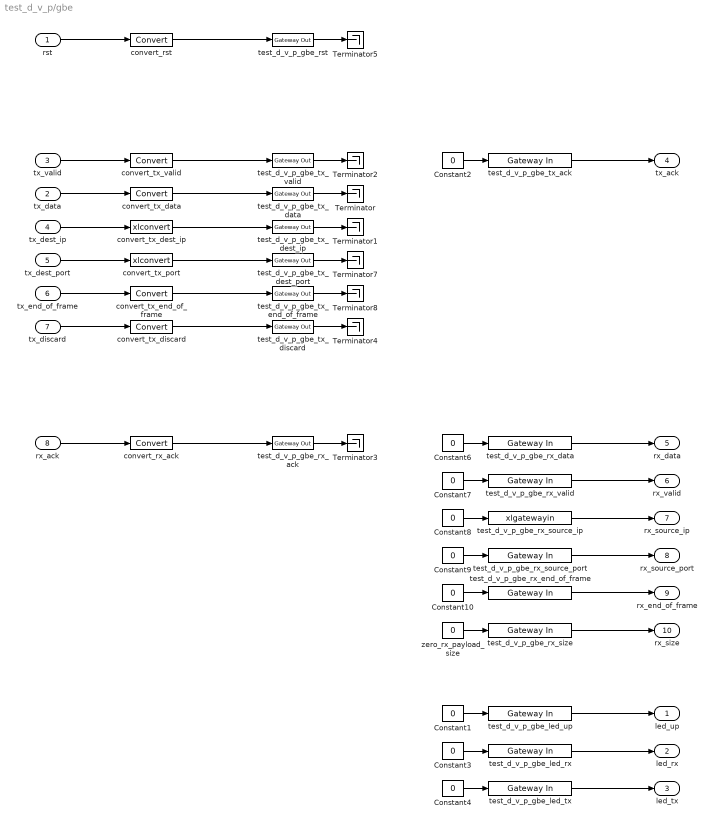
== system test_d_v_p/gbe ==
  rst : Inport  Port=1  LatchInput=off
  tx_data : Inport  Port=2  LatchInput=off
  tx_valid : Inport  Port=3  LatchInput=off
  tx_dest_ip : Inport  Port=4  LatchInput=off
  tx_dest_port : Inport  Port=5  LatchInput=off
  tx_end_of_frame : Inport  Port=6  LatchInput=off
  tx_discard : Inport  Port=7  LatchInput=off
  rx_ack : Inport  Port=8  LatchInput=off
  Constant{1..4,6..10} (9 alike) : Constant  Value=0
  Terminator{,1..5,7..8} (8 alike) : Terminator
  convert_rst : xbsIndex_r3/Convert  arith_type=Boolean  n_bits=64  bin_pt=0  quantization=Truncate  overflow=Wrap  latency=0  explicit_period=off  period=1  dbl_ovrd=off  show_param=off  inserted_by_tool=off  pipeline=off
      settings: xl_area=[0, 0, 0, 0, 0, 0, 0]
  convert_rx_ack : xbsIndex_r3/Convert  arith_type=Boolean  n_bits=64  bin_pt=0  quantization=Truncate  overflow=Wrap  latency=0  explicit_period=off  period=1  dbl_ovrd=off  show_param=off  inserted_by_tool=off  pipeline=off
      settings: xl_area=[0, 0, 0, 0, 0, 0, 0]
  convert_tx_data : xbsIndex_r3/Convert  arith_type=Unsigned  n_bits=64  bin_pt=0  quantization=Truncate  overflow=Wrap  latency=0  explicit_period=off  period=1  dbl_ovrd=off  show_param=off  inserted_by_tool=off  pipeline=off
      settings: xl_area=[0, 0, 0, 0, 0, 0, 0]
  convert_tx_dest_ip : S-Function  AncestorBlock=xbsIndex_r3/Convert  FunctionName=xlconvert  Parameters=sfcn_mwsv__  mask(Xilinx Converter Block){arith_type=Unsigned, n_bits=32, bin_pt=0, quantization=Truncate, overflow=Wrap, latency=0, explicit_period=off, period=1, dbl_ovrd=off, show_param=off, inserted_by_tool=off, pipeline=off, xl_area=[0, 0, 0, 0, 0, 0, 0], xl_use_area=off}
      mask prompts: arith_type "Output Type"; n_bits "Number of Bits"; bin_pt "Binary Point"; quantization "Quantization Behavior"; overflow "Overflow Behavior"; explicit_period "Use Explicit Sample Period"; period "Sample Period"; dbl_ovrd "Override with Doubles"; show_param "---------------------- Show Implementation Parameters -----------------------------------------------------------------------------------"; inserted_by_tool "Hidden Parameter:  inserted_by_tool"; pipeline "Pipeline to Greatest Extent Possible"; xl_area "FPGA Area [Slices, FFs, BRAMs, LUTs, IOBs, Emb. Mults, TBUFs]"; xl_use_area "Use Area Above For Estimation"
      mask help:
      | Type conversion block. The input is presented at the output after quantization and overflow effects.
      |
      | Hardware notes: Additional hardware is used when rounding or saturation is selected and output width is less than the input width.
      mask init:
      | [designRoot, family, part, speed, package, simulinkPeriod, sysclkPeriod, dbl_ovrd, trimVbit] = xlSysgenSettings(gcb,1,1);
      | if (arith_type==1)
      |   bool = 1;
      | else
      |   bool = 0;
      |   arith_type = arith_type-1;
      | end
      | zstr=''; zpstr='';
      | if latency > 0
      |   zstr = 'z';
      |   zpstr = sprintf('-%d', latency);
      | end
      | [bg,fg] = xlcmap('XBlock',dbl_ovrd);
      | if (inserted_by_tool)
      |   bg = [1.00 0.50 0.25];
      | end
      | iPos = get_param(gcb,'Position');
      | iWidth=iPos(3)-iPos(1); iHeight=iPos(4)-iPos(2);
      | iCx=iWidth/2;
      | iCy=iHeight/2;
      | [logoX, logoY] = xlogo(iPos);
      | zstrx = 0.45*iWidth-11; if (zstrx<3) zstrx=3; end
      | zstry = 0.36*iHeight-7; if (zstry<3) zstry=3; end
      | 
      | 
      | % one time added for param list
      | dblOvrd = dbl_ovrd;
      | precision0 = 2;
      | z0 = [n_bits bin_pt arith_type quantization overflow];
      | explicitClk = explicit_period;
      | 
      | 
      | % just pass everything to s-function
      | sfcn_mwsv__ = get_param(gcb, 'MaskWSVariables');
      mask Help: eval('xlWeb(xlhtmldoclink(''Convert''))');
      mask StyleString: popup(Boolean|Unsigned|Signed  (2's comp)),edit,edit,popup(Truncate|Round  (unbiased: +/- Inf)|Round  (unbiased: Even Values)),popup(Wrap|Saturate|Error),edit,checkbox,edit,checkbox,checkbox,checkbox,checkbox,edit,checkbox
      mask CallbackString: xlconvertCallback||||||xlMagicCallback|||xlShowIPCallback||||
      mask Display:
      | patch([0 iWidth iWidth 0],[0 0 iHeight iHeight] , bg);
      | patch(logoX,logoY , fg);
      | text(zstrx,zstry,zstr);
      | text(zstrx+5,zstry+5,zpstr);
      | port_label('output',1,'cast');
      | plot([0 0 iWidth iWidth 0], [0 iHeight iHeight 0 0]);
  convert_tx_discard : xbsIndex_r3/Convert  arith_type=Boolean  n_bits=1  bin_pt=0  quantization=Truncate  overflow=Wrap  latency=0  explicit_period=off  period=1  dbl_ovrd=off  show_param=off  inserted_by_tool=off  pipeline=off
      settings: xl_area=[0, 0, 0, 0, 0, 0, 0]
  convert_tx_end_of_frame : xbsIndex_r3/Convert  arith_type=Boolean  n_bits=1  bin_pt=0  quantization=Truncate  overflow=Wrap  latency=0  explicit_period=off  period=1  dbl_ovrd=off  show_param=off  inserted_by_tool=off  pipeline=off
      settings: xl_area=[0, 0, 0, 0, 0, 0, 0]
  convert_tx_port : S-Function  AncestorBlock=xbsIndex_r3/Convert  FunctionName=xlconvert  Parameters=sfcn_mwsv__  mask(Xilinx Converter Block){arith_type=Unsigned, n_bits=16, bin_pt=0, quantization=Truncate, overflow=Wrap, latency=0, explicit_period=off, period=1, dbl_ovrd=off, show_param=off, inserted_by_tool=off, pipeline=off, xl_area=[0, 0, 0, 0, 0, 0, 0], xl_use_area=off}
      mask prompts: arith_type "Output Type"; n_bits "Number of Bits"; bin_pt "Binary Point"; quantization "Quantization Behavior"; overflow "Overflow Behavior"; explicit_period "Use Explicit Sample Period"; period "Sample Period"; dbl_ovrd "Override with Doubles"; show_param "---------------------- Show Implementation Parameters -----------------------------------------------------------------------------------"; inserted_by_tool "Hidden Parameter:  inserted_by_tool"; pipeline "Pipeline to Greatest Extent Possible"; xl_area "FPGA Area [Slices, FFs, BRAMs, LUTs, IOBs, Emb. Mults, TBUFs]"; xl_use_area "Use Area Above For Estimation"
      mask help:
      | Type conversion block. The input is presented at the output after quantization and overflow effects.
      |
      | Hardware notes: Additional hardware is used when rounding or saturation is selected and output width is less than the input width.
      mask init: same as test_d_v_p/gbe/convert_tx_dest_ip
      mask Help: eval('xlWeb(xlhtmldoclink(''Convert''))');
      mask StyleString: popup(Boolean|Unsigned|Signed  (2's comp)),edit,edit,popup(Truncate|Round  (unbiased: +/- Inf)|Round  (unbiased: Even Values)),popup(Wrap|Saturate|Error),edit,checkbox,edit,checkbox,checkbox,checkbox,checkbox,edit,checkbox
      mask CallbackString: xlconvertCallback||||||xlMagicCallback|||xlShowIPCallback||||
      mask Display:
      | patch([0 iWidth iWidth 0],[0 0 iHeight iHeight] , bg);
      | patch(logoX,logoY , fg);
      | text(zstrx,zstry,zstr);
      | text(zstrx+5,zstry+5,zpstr);
      | port_label('output',1,'cast');
      | plot([0 0 iWidth iWidth 0], [0 iHeight iHeight 0 0]);
  convert_tx_valid : xbsIndex_r3/Convert  arith_type=Boolean  n_bits=1  bin_pt=0  quantization=Truncate  overflow=Wrap  latency=0  explicit_period=off  period=1  dbl_ovrd=off  show_param=off  inserted_by_tool=off  pipeline=off
      settings: xl_area=[0, 0, 0, 0, 0, 0, 0]
  test_d_v_p_gbe_led_rx : xbsIndex_r3/Gateway In  arith_type=Boolean  n_bits=1  bin_pt=0  quantization=Truncate  overflow=Wrap  period=1  timing_constraint=None  locs_specified=off  LOCs={}  needs_fixed_name=off  dbl_ovrd=off  show_param=off
      settings: xl_area=[0, 0, 0, 0, 0, 0, 0]
  test_d_v_p_gbe_led_tx : xbsIndex_r3/Gateway In  arith_type=Boolean  n_bits=1  bin_pt=0  quantization=Truncate  overflow=Wrap  period=1  timing_constraint=None  locs_specified=off  LOCs={}  needs_fixed_name=off  dbl_ovrd=off  show_param=off
      settings: xl_area=[0, 0, 0, 0, 0, 0, 0]
  test_d_v_p_gbe_led_up : xbsIndex_r3/Gateway In  arith_type=Boolean  n_bits=1  bin_pt=0  quantization=Truncate  overflow=Wrap  period=1  timing_constraint=None  locs_specified=off  LOCs={}  needs_fixed_name=off  dbl_ovrd=off  show_param=off
      settings: xl_area=[0, 0, 0, 0, 0, 0, 0]
  test_d_v_p_gbe_rst : xbsIndex_r3/Gateway Out  output_type=Double  nbits=8  bin_pt=6  arith_type=Boolean  quantization=Truncate  overflow=Wrap  hdl_port=on  timing_constraint=None  locs_specified=off  LOCs={}  needs_fixed_name=off  show_param=off
      settings: xl_area=[0, 0, 0, 0, 0, 0, 0]
  test_d_v_p_gbe_rx_ack : xbsIndex_r3/Gateway Out  output_type=Double  nbits=8  bin_pt=6  arith_type=Boolean  quantization=Truncate  overflow=Wrap  hdl_port=on  timing_constraint=None  locs_specified=off  LOCs={}  needs_fixed_name=off  show_param=off
      settings: xl_area=[0, 0, 0, 0, 0, 0, 0]
  test_d_v_p_gbe_rx_data : xbsIndex_r3/Gateway In  arith_type=Unsigned  n_bits=64  bin_pt=0  quantization=Truncate  overflow=Wrap  period=1  timing_constraint=None  locs_specified=off  LOCs={}  needs_fixed_name=off  dbl_ovrd=off  show_param=off
      settings: xl_area=[0, 0, 0, 0, 0, 0, 0]
  test_d_v_p_gbe_rx_end_of_frame : xbsIndex_r3/Gateway In  arith_type=Boolean  n_bits=1  bin_pt=0  quantization=Truncate  overflow=Wrap  period=1  timing_constraint=None  locs_specified=off  LOCs={}  needs_fixed_name=off  dbl_ovrd=off  show_param=off
      settings: xl_area=[0, 0, 0, 0, 0, 0, 0]
  test_d_v_p_gbe_rx_size : xbsIndex_r3/Gateway In  arith_type=Unsigned  n_bits=16  bin_pt=0  quantization=Truncate  overflow=Wrap  period=1  timing_constraint=None  locs_specified=off  LOCs={}  needs_fixed_name=off  dbl_ovrd=off  show_param=off
      settings: xl_area=[0, 0, 0, 0, 0, 0, 0]
  test_d_v_p_gbe_rx_source_ip : S-Function  AncestorBlock=xbsIndex_r3/Gateway In  FunctionName=xlgatewayin  Parameters="arith_type, n_bits, bin_pt, quantization, overflow,  gcb, period, dbl_ovrd, locs_specified, LOCs, timing_constraint, simulinkPeriod, designRoot, 0"  mask(Xilinx Gateway In){arith_type=Unsigned, n_bits=32, bin_pt=0, quantization=Truncate, overflow=Wrap, period=1, timing_constraint=None, locs_specified=off, LOCs={}, needs_fixed_name=off, dbl_ovrd=off, show_param=off, xl_area=[0, 0, 0, 0, 0, 0, 0], xl_use_area=off}
      mask prompts: arith_type "Output Data Type"; n_bits "Number of Bits"; bin_pt "Binary Point"; period "Sample Period"; timing_constraint "IOB Timing Constraint"; locs_specified "Specify IOB Location Constraints"; LOCs "IOB Pad Locations (specify as cell array {'MSB', ..., 'LSB'})"; needs_fixed_name "Do Not Prepend Hierarchy to Port Name"; dbl_ovrd "Override with Double"; show_param "---------------------- Show Implementation Parameters -----------------------------------------------------------------------------------"; xl_area "FPGA Area [Slices, FFs, BRAMs, LUTs, IOBs, Emb. Mults, TBUFs]"; xl_use_area "Use Area Above For Estimation"
      mask help:
      | Gateway in block.  Converts inputs of type Simulink integer, double and fixed point to  Xilinx fixed point type.
      |
      | Hardware notes:  In hardware these blocks become top level input ports.
      mask init:
      | [designRoot, family, part, speed, package, simulinkPeriod, sysclkPeriod, dbl_ovrd, trimVbit] = xlSysgenSettings(gcb,1,0);
      | trimVbit = 1;
      | [bg,fg] = xlcmap('IO',dbl_ovrd);
      | iPos = get_param(gcb,'Position');
      | iWidth=iPos(3)-iPos(1); iHeight=iPos(4)-iPos(2);
      | iCx=iWidth/2;
      | iCy=iHeight/2;
      | [logoX, logoY] = xlogo(iPos);
      mask Help: eval('xlWeb(xlhtmldoclink(''Gateway In''))');
      mask StyleString: popup(Boolean|Unsigned|Signed  (2's comp)),edit,edit,popup(Truncate|Round  (unbiased: +/- Inf)),popup(Wrap|Saturate|Flag as Error),edit,popup(None|Data Rate|Data Rate;  Set 'FAST' Attribute),checkbox,edit,checkbox,checkbox,checkbox,edit,checkbox
      mask CallbackString: xlgatewayinCallback|||||||xlgatewayinCallback||||xlShowIPCallback||
      mask Display:
      | patch([0 iWidth iWidth 0],[0 0 iHeight iHeight] , bg);
      | patch(logoX,logoY , fg);
      | port_label('input',1,'dbl');
      | port_label('output',1,'fpt');
      | 
      | ;plot([0 0 iWidth iWidth 0], [0 iHeight iHeight 0 0]);
  test_d_v_p_gbe_rx_source_port : xbsIndex_r3/Gateway In  arith_type=Unsigned  n_bits=16  bin_pt=0  quantization=Truncate  overflow=Wrap  period=1  timing_constraint=None  locs_specified=off  LOCs={}  needs_fixed_name=off  dbl_ovrd=off  show_param=off
      settings: xl_area=[0, 0, 0, 0, 0, 0, 0]
  test_d_v_p_gbe_rx_valid : xbsIndex_r3/Gateway In  arith_type=Boolean  n_bits=1  bin_pt=0  quantization=Truncate  overflow=Wrap  period=1  timing_constraint=None  locs_specified=off  LOCs={}  needs_fixed_name=off  dbl_ovrd=off  show_param=off
      settings: xl_area=[0, 0, 0, 0, 0, 0, 0]
  test_d_v_p_gbe_tx_ack : xbsIndex_r3/Gateway In  arith_type=Boolean  n_bits=1  bin_pt=0  quantization=Truncate  overflow=Wrap  period=1  timing_constraint=None  locs_specified=off  LOCs={}  needs_fixed_name=off  dbl_ovrd=off  show_param=off
      settings: xl_area=[0, 0, 0, 0, 0, 0, 0]
  test_d_v_p_gbe_tx_data : xbsIndex_r3/Gateway Out  output_type=Double  nbits=8  bin_pt=6  arith_type=Boolean  quantization=Truncate  overflow=Wrap  hdl_port=on  timing_constraint=None  locs_specified=off  LOCs={}  needs_fixed_name=off  show_param=off
      settings: xl_area=[0, 0, 0, 0, 0, 0, 0]
  test_d_v_p_gbe_tx_dest_ip : xbsIndex_r3/Gateway Out  output_type=Double  nbits=8  bin_pt=6  arith_type=Boolean  quantization=Truncate  overflow=Wrap  hdl_port=on  timing_constraint=None  locs_specified=off  LOCs={}  needs_fixed_name=off  show_param=off
      settings: xl_area=[0, 0, 0, 0, 0, 0, 0]
  test_d_v_p_gbe_tx_dest_port : xbsIndex_r3/Gateway Out  output_type=Double  nbits=8  bin_pt=6  arith_type=Boolean  quantization=Truncate  overflow=Wrap  hdl_port=on  timing_constraint=None  locs_specified=off  LOCs={}  needs_fixed_name=off  show_param=off
      settings: xl_area=[0, 0, 0, 0, 0, 0, 0]
  test_d_v_p_gbe_tx_discard : xbsIndex_r3/Gateway Out  output_type=Double  nbits=8  bin_pt=6  arith_type=Boolean  quantization=Truncate  overflow=Wrap  hdl_port=on  timing_constraint=None  locs_specified=off  LOCs={}  needs_fixed_name=off  show_param=off
      settings: xl_area=[0, 0, 0, 0, 0, 0, 0]
  test_d_v_p_gbe_tx_end_of_frame : xbsIndex_r3/Gateway Out  output_type=Double  nbits=8  bin_pt=6  arith_type=Boolean  quantization=Truncate  overflow=Wrap  hdl_port=on  timing_constraint=None  locs_specified=off  LOCs={}  needs_fixed_name=off  show_param=off
      settings: xl_area=[0, 0, 0, 0, 0, 0, 0]
  test_d_v_p_gbe_tx_valid : xbsIndex_r3/Gateway Out  output_type=Double  nbits=8  bin_pt=6  arith_type=Boolean  quantization=Truncate  overflow=Wrap  hdl_port=on  timing_constraint=None  locs_specified=off  LOCs={}  needs_fixed_name=off  show_param=off
      settings: xl_area=[0, 0, 0, 0, 0, 0, 0]
  zero_rx_payload_size : Constant  Value=0
  led_up : Outport
  led_rx : Outport  Port=2
  led_tx : Outport  Port=3
  tx_ack : Outport  Port=4
  rx_data : Outport  Port=5
  rx_valid : Outport  Port=6
  rx_source_ip : Outport  Port=7
  rx_source_port : Outport  Port=8
  rx_end_of_frame : Outport  Port=9
  rx_size : Outport  Port=10
  wires:
  test_d_v_p_gbe_tx_discard/1 -> Terminator4/1
  convert_tx_discard/1 -> test_d_v_p_gbe_tx_discard/1
  tx_discard/1 -> convert_tx_discard/1
  test_d_v_p_gbe_rx_size/1 -> rx_size/1
  zero_rx_payload_size/1 -> test_d_v_p_gbe_rx_size/1
  test_d_v_p_gbe_led_tx/1 -> led_tx/1
  Constant4/1 -> test_d_v_p_gbe_led_tx/1
  test_d_v_p_gbe_led_rx/1 -> led_rx/1
  Constant3/1 -> test_d_v_p_gbe_led_rx/1
  test_d_v_p_gbe_led_up/1 -> led_up/1
  Constant1/1 -> test_d_v_p_gbe_led_up/1
  test_d_v_p_gbe_rx_end_of_frame/1 -> rx_end_of_frame/1
  Constant10/1 -> test_d_v_p_gbe_rx_end_of_frame/1
  test_d_v_p_gbe_rx_source_port/1 -> rx_source_port/1
  Constant9/1 -> test_d_v_p_gbe_rx_source_port/1
  Constant8/1 -> test_d_v_p_gbe_rx_source_ip/1
  test_d_v_p_gbe_rx_source_ip/1 -> rx_source_ip/1
  test_d_v_p_gbe_tx_end_of_frame/1 -> Terminator8/1
  convert_tx_end_of_frame/1 -> test_d_v_p_gbe_tx_end_of_frame/1
  tx_end_of_frame/1 -> convert_tx_end_of_frame/1
  test_d_v_p_gbe_tx_dest_port/1 -> Terminator7/1
  convert_tx_port/1 -> test_d_v_p_gbe_tx_dest_port/1
  tx_dest_port/1 -> convert_tx_port/1
  test_d_v_p_gbe_rst/1 -> Terminator5/1
  convert_rst/1 -> test_d_v_p_gbe_rst/1
  rst/1 -> convert_rst/1
  test_d_v_p_gbe_rx_valid/1 -> rx_valid/1
  Constant7/1 -> test_d_v_p_gbe_rx_valid/1
  test_d_v_p_gbe_rx_ack/1 -> Terminator3/1
  Constant6/1 -> test_d_v_p_gbe_rx_data/1
  Constant2/1 -> test_d_v_p_gbe_tx_ack/1
  test_d_v_p_gbe_tx_valid/1 -> Terminator2/1
  test_d_v_p_gbe_tx_dest_ip/1 -> Terminator1/1
  test_d_v_p_gbe_tx_data/1 -> Terminator/1
  test_d_v_p_gbe_tx_ack/1 -> tx_ack/1
  convert_tx_valid/1 -> test_d_v_p_gbe_tx_valid/1
  tx_valid/1 -> convert_tx_valid/1
  convert_tx_dest_ip/1 -> test_d_v_p_gbe_tx_dest_ip/1
  tx_dest_ip/1 -> convert_tx_dest_ip/1
  convert_tx_data/1 -> test_d_v_p_gbe_tx_data/1
  tx_data/1 -> convert_tx_data/1
  test_d_v_p_gbe_rx_data/1 -> rx_data/1
  convert_rx_ack/1 -> test_d_v_p_gbe_rx_ack/1
  rx_ack/1 -> convert_rx_ack/1

== system test_d_v_p/pulse_ext ==
  in : Inport  Port=1  LatchInput=off
  Constant : xbsIndex_r3/Constant  const=1  equ=P=C  arith_type=Boolean  n_bits=1  bin_pt=0  opselect=C  inp2=PCIN>>17  opr=+  inp1=P  carry=CIN  iostate=0  explicit_period=off  period=1  dbl_ovrd=off
  Constant17 : xbsIndex_r3/Constant  const=pulse_len  equ=P=C  arith_type=Unsigned  n_bits=bits  bin_pt=0  opselect=C  inp2=PCIN>>17  opr=+  inp1=P  carry=CIN  iostate=0  explicit_period=on  period=1  dbl_ovrd=off
  Relational1 : xbsIndex_r3/Relational  mode=a<b  latency=0  explicit_period=off  period=1  en=off  dbl_ovrd=off  show_param=off
      settings: xl_area=[0, 0, 0, 0, 0, 0, 0]
  Terminator : Terminator
  freeze_cntr : Subsystem  mask{CounterBits=bits}
      mask prompts: CounterBits "Counter Length (2^?)"
  posedge : Subsystem  Tag=Rising Edge Detector
  out : Outport
  wires:
  Constant/1 -> freeze_cntr/1(en)
  freeze_cntr/2(we) -> Terminator/1
  freeze_cntr/1(addr) -> Relational1/1
  posedge/1(Out) -> freeze_cntr/2(rst)
  Constant17/1 -> Relational1/2
  Relational1/1 -> out/1
  in/1 -> posedge/1(In)
